simulink model "Model_RL_s"  (R2023a)
settings: Solver=VariableStepAuto  StartTime=0.0  StopTime=20  MaxStep=0.002  RelTol=1e-6
StopFcn:
  | save_run_results('RL', 'manual_run')
values from neighbouring files (symbols this model uses):
  C_r = maskInitContext.MaskWorkspace.get('C_r')    [Mask_bike.m]
  F_zf = m_ * g_ * l_r_ / (l_f_ + l_r_)    [load_derived.m]
  F_zr = m_ * g_ * l_f_ / (l_f_ + l_r_)    [load_derived.m]
  l_f = maskInitContext.MaskWorkspace.get('l_f')    [Mask_Pacejka.m]    (also in Mask_bike.m)
  l_r = maskInitContext.MaskWorkspace.get('l_r')    [Mask_bike.m]
  m = maskInitContext.MaskWorkspace.get('m')    [Mask_bike.m]
  Tdref_ay_bp_ms2 = raw.fine.ay_breakpoints_g(:)' * 9.81    [load_ref.m]
  Tdref_table = raw.fine.table_Nm'    [load_ref.m]
  Tdref_v_bp_ms = raw.fine.v_breakpoints_kmh(:)' / 3.6    [load_ref.m]
undefined symbols (not defined in the file or in its folder): c, C, C_alpha_f, C_col, E, e_c, Iz, J_col, K, n_st, noise_seed_a_y, noise_seed_gamma, noise_seed_T_s, noise_seed_theta1, noise_seed_theta2_dot, noise_seed_v, noise_var_a_y, noise_var_gamma, noise_var_T_s, noise_var_theta1, noise_var_theta2_dot, noise_var_v, rl_done_eT, rl_hist_stride, rl_I_decay, rl_I_gain, rl_I_in, rl_obs_gain, rl_reward_par, rl_Ta_gain, rl_Ts, rl_use_agent, sens_Tupd_a_y, sens_Tupd_gamma, sens_Tupd_T_s, sens_Tupd_theta1, sens_Tupd_theta2_dot, sens_Tupd_v, sensors_on, t_0, T_f, Tamax_table, Tamax_v_bp_ms
libraries: rllib x1
settings Model: Creator=Tan_Tram  LastModifiedBy=Tan_Tram
settings DataIOCC: ReturnWorkspaceOutputs=off

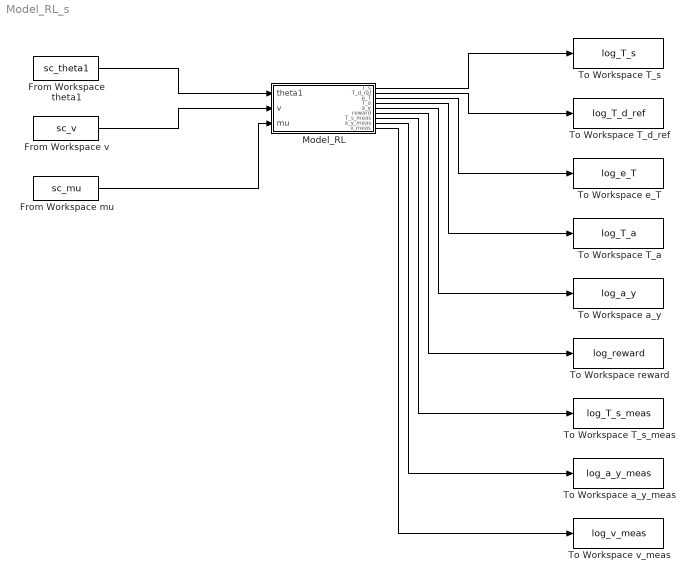
== system Model_RL_s ==
  From Workspace mu : FromWorkspace  VariableName=sc_mu  OutputAfterFinalValue=Holding final value
  From Workspace theta1 : FromWorkspace  VariableName=sc_theta1  OutputAfterFinalValue=Holding final value
  From Workspace v : FromWorkspace  VariableName=sc_v  OutputAfterFinalValue=Holding final value
  Model_RL : Subsystem
  To Workspace T_a : ToWorkspace  VariableName=log_T_a  SaveFormat=Timeseries  SampleTime=-1
  To Workspace T_d_ref : ToWorkspace  VariableName=log_T_d_ref  SaveFormat=Timeseries  SampleTime=-1
  To Workspace T_s : ToWorkspace  VariableName=log_T_s  SaveFormat=Timeseries  SampleTime=-1
  To Workspace T_s_meas : ToWorkspace  VariableName=log_T_s_meas  SaveFormat=Timeseries  SampleTime=-1
  To Workspace a_y : ToWorkspace  VariableName=log_a_y  SaveFormat=Timeseries  SampleTime=-1
  To Workspace a_y_meas : ToWorkspace  VariableName=log_a_y_meas  SaveFormat=Timeseries  SampleTime=-1
  To Workspace e_T : ToWorkspace  VariableName=log_e_T  SaveFormat=Timeseries  SampleTime=-1
  To Workspace reward : ToWorkspace  VariableName=log_reward  SaveFormat=Timeseries  SampleTime=-1
  To Workspace v_meas : ToWorkspace  VariableName=log_v_meas  SaveFormat=Timeseries  SampleTime=-1
  wires:
  From Workspace theta1/1 -> Model_RL/1(theta1)
  From Workspace v/1 -> Model_RL/2(v)
  From Workspace mu/1 -> Model_RL/3(mu)
  Model_RL/1(T_s) -> To Workspace T_s/1
  Model_RL/2(T_d_ref) -> To Workspace T_d_ref/1
  Model_RL/3(e_T) -> To Workspace e_T/1
  Model_RL/4(T_a) -> To Workspace T_a/1
  Model_RL/5(a_y) -> To Workspace a_y/1
  Model_RL/6(reward) -> To Workspace reward/1
  Model_RL/7(T_s_meas) -> To Workspace T_s_meas/1
  Model_RL/8(a_y_meas) -> To Workspace a_y_meas/1
  Model_RL/9(v_meas) -> To Workspace v_meas/1

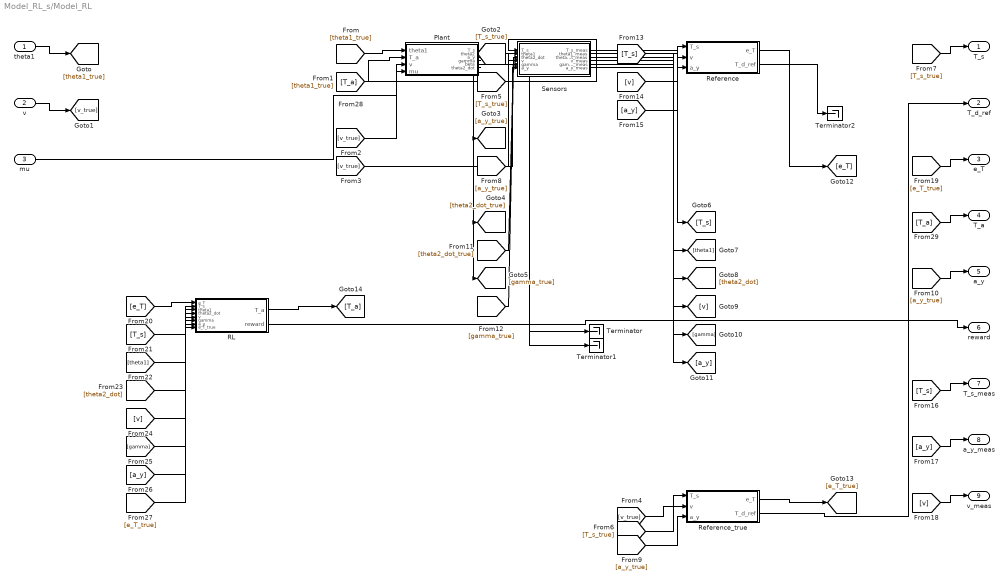
== system Model_RL_s/Model_RL ==
  theta1 : Inport
  v : Inport  Port=2
  mu : Inport  Port=3
  Plant : Subsystem
  RL : Subsystem
  Reference : Subsystem
  Reference_true : Subsystem
  Sensors : Subsystem
  Terminator : Terminator
  Terminator1 : Terminator
  Terminator2 : Terminator
  T_s : Outport
  T_d_ref : Outport  Port=2
  e_T : Outport  Port=3
  T_a : Outport  Port=4
  a_y : Outport  Port=5
  reward : Outport  Port=6
  T_s_meas : Outport  Port=7
  a_y_meas : Outport  Port=8
  v_meas : Outport  Port=9
  wires:
  theta1/1 -> [theta1_true]
  [theta1_true] -> Plant/1(theta1)
  [theta1_true] -> Sensors/2(theta1)
  v/1 -> [v_true]
  [v_true] -> Plant/3(v)
  [v_true] -> Sensors/4(v)
  [v_true] -> Reference_true/2(v)
  mu/1 -> Plant/4(mu)
  Plant/1(T_s) -> [T_s_true]
  [T_s_true] -> Sensors/1(T_s)
  [T_s_true] -> Reference_true/1(T_s)
  [T_s_true] -> T_s/1
  Plant/3(a_y) -> [a_y_true]
  [a_y_true] -> Sensors/6(a_y)
  [a_y_true] -> Reference_true/3(a_y)
  [a_y_true] -> a_y/1
  Plant/6(theta2_dot) -> [theta2_dot_true]
  [theta2_dot_true] -> Sensors/3(theta2_dot)
  Plant/4(gamma) -> [gamma_true]
  [gamma_true] -> Sensors/5(gamma)
  Plant/2(theta2) -> Terminator/1
  Plant/5(beta) -> Terminator1/1
  Sensors/1(T_s_meas) -> [T_s]
  Sensors/2(theta1_meas) -> [theta1]
  Sensors/3(theta2_dot_meas) -> [theta2_dot]
  Sensors/4(v_meas) -> [v]
  Sensors/5(gamma_meas) -> [gamma]
  Sensors/6(a_y_meas) -> [a_y]
  [T_s] -> Reference/1(T_s)
  [v] -> Reference/2(v)
  [a_y] -> Reference/3(a_y)
  [T_s] -> T_s_meas/1
  [a_y] -> a_y_meas/1
  [v] -> v_meas/1
  Reference/1(e_T) -> [e_T]
  Reference/2(T_d_ref) -> Terminator2/1
  Reference_true/1(e_T) -> [e_T_true]
  [e_T_true] -> e_T/1
  Reference_true/2(T_d_ref) -> T_d_ref/1
  [e_T] -> RL/1(e_T)
  [T_s] -> RL/2(T_s)
  [theta1] -> RL/3(theta1)
  [theta2_dot] -> RL/4(theta2_dot)
  [v] -> RL/5(v)
  [gamma] -> RL/6(gamma)
  [a_y] -> RL/7(a_y)
  [e_T_true] -> RL/8(e_T_true)
  RL/1(T_a) -> [T_a]
  [T_a] -> Plant/2(T_a)
  [T_a] -> T_a/1
  RL/2(reward) -> reward/1

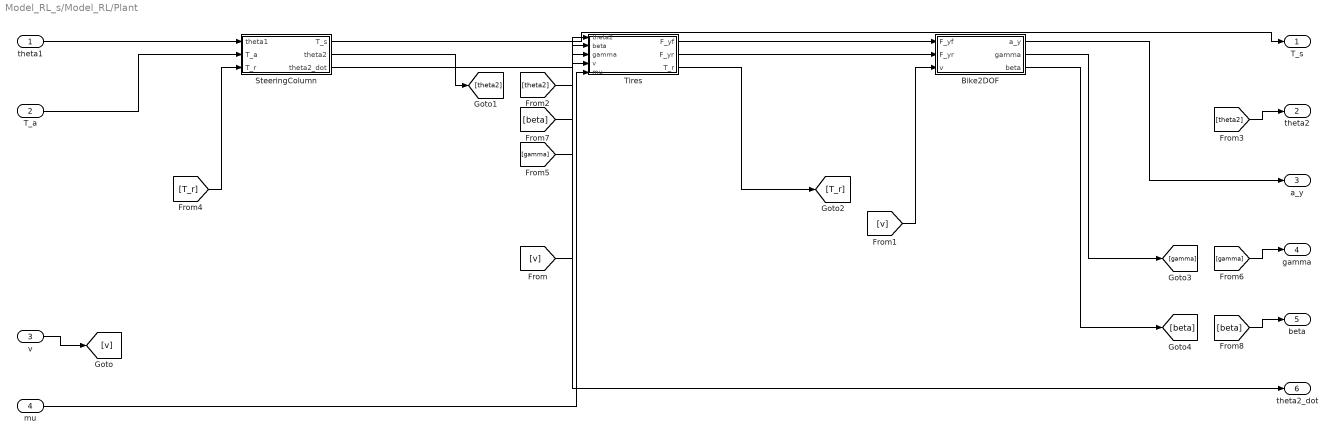
== system Model_RL_s/Model_RL/Plant ==
  theta1 : Inport
  T_a : Inport  Port=2
  v : Inport  Port=3
  mu : Inport  Port=4
  Bike2DOF : Subsystem
  SteeringColumn : Subsystem
  Tires : Subsystem
  T_s : Outport
  theta2 : Outport  Port=2
  a_y : Outport  Port=3
  gamma : Outport  Port=4
  beta : Outport  Port=5
  theta2_dot : Outport  Port=6
  wires:
  [beta] -> beta/1
  [beta] -> Tires/2(beta)
  Bike2DOF/3(beta) -> [beta]
  [gamma] -> gamma/1
  [gamma] -> Tires/3(gamma)
  Bike2DOF/2(gamma) -> [gamma]
  [T_r] -> SteeringColumn/3(T_r)
  Tires/3(T_r) -> [T_r]
  [theta2] -> theta2/1
  [theta2] -> Tires/1(theta2)
  SteeringColumn/2(theta2) -> [theta2]
  [v] -> Bike2DOF/3(v)
  [v] -> Tires/4(v)
  v/1 -> [v]
  SteeringColumn/3(theta2_dot) -> theta2_dot/1
  Bike2DOF/1(a_y) -> a_y/1
  SteeringColumn/1(T_s) -> T_s/1
  Tires/2(F_yr) -> Bike2DOF/2(F_yr)
  Tires/1(F_yf) -> Bike2DOF/1(F_yf)
  mu/1 -> Tires/5(mu)
  T_a/1 -> SteeringColumn/2(T_a)
  theta1/1 -> SteeringColumn/1(theta1)

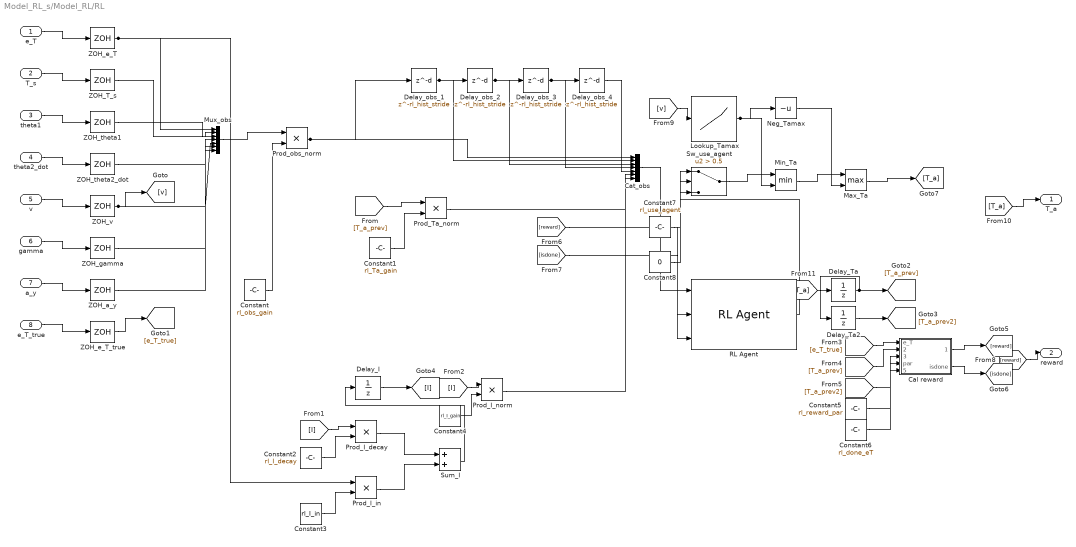
== system Model_RL_s/Model_RL/RL ==
  e_T : Inport
  T_s : Inport  Port=2
  theta1 : Inport  Port=3
  theta2_dot : Inport  Port=4
  v : Inport  Port=5
  gamma : Inport  Port=6
  a_y : Inport  Port=7
  e_T_true : Inport  Port=8
  Cal reward : MATLAB Function  TreatAsAtomicUnit=on
  Cat_obs : Concatenate  NumInputs=7
  Constant : Constant  Value=rl_obs_gain
  Constant1 : Constant  Value=rl_Ta_gain
  Constant2 : Constant  Value=rl_I_decay
  Constant3 : Constant  Value=rl_I_in
  Constant4 : Constant  Value=rl_I_gain
  Constant5 : Constant  Value=rl_reward_par
  Constant6 : Constant  Value=rl_done_eT
  Constant7 : Constant  Value=rl_use_agent
  Constant8 : Constant  Value=0
  Delay_I : UnitDelay  SampleTime=rl_Ts  HasFrameUpgradeWarning=on
  Delay_Ta : UnitDelay  SampleTime=rl_Ts  HasFrameUpgradeWarning=on
  Delay_Ta2 : UnitDelay  SampleTime=rl_Ts  HasFrameUpgradeWarning=on
  Delay_obs_{1..4} (4 alike) : Delay  DelayLength=rl_hist_stride  InitialCondition=0  SampleTime=rl_Ts
  Lookup_Tamax : Lookup_n-D  NumberOfTableDimensions=1  BreakpointsForDimension1=Tamax_v_bp_ms  Table=Tamax_table  ExtrapMethod=Clip  InternalRulePriority=Speed  RndMeth=Simplest
  Max_Ta : MinMax  Function=max  Inputs=2
  Min_Ta : MinMax  Inputs=2
  Mux_obs : Mux  Inputs=7
  Neg_Tamax : UnaryMinus
  Prod_I_decay : Product  Inputs=**
  Prod_I_in : Product  Inputs=**
  Prod_I_norm : Product  Inputs=**
  Prod_Ta_norm : Product  Inputs=**
  Prod_obs_norm : Product  Inputs=**
  RL Agent : rllib/RL Agent  Agent=rl_agent  ExternalActionAsInput=off  ProvideLastAction=off  ProvideCumRwd=off  TreatAsDirectFeedthrough=on  UseStrictObservationDataTypes=off
  Sum_I : Sum
  Sw_use_agent : Switch  Criteria=u2 > Threshold  Threshold=0.5  SaturateOnIntegerOverflow=off  InputSameDT=off
  ZOH_T_s : ZeroOrderHold  SampleTime=rl_Ts
  ZOH_a_y : ZeroOrderHold  SampleTime=rl_Ts
  ZOH_e_T : ZeroOrderHold  SampleTime=rl_Ts
  ZOH_e_T_true : ZeroOrderHold  SampleTime=rl_Ts
  ZOH_gamma : ZeroOrderHold  SampleTime=rl_Ts
  ZOH_theta1 : ZeroOrderHold  SampleTime=rl_Ts
  ZOH_theta2_dot : ZeroOrderHold  SampleTime=rl_Ts
  ZOH_v : ZeroOrderHold  SampleTime=rl_Ts
  T_a : Outport
  reward : Outport  Port=2
  wires:
  e_T/1 -> ZOH_e_T/1
  T_s/1 -> ZOH_T_s/1
  theta1/1 -> ZOH_theta1/1
  theta2_dot/1 -> ZOH_theta2_dot/1
  v/1 -> ZOH_v/1
  ZOH_v/1 -> [v], Mux_obs/5
  gamma/1 -> ZOH_gamma/1
  a_y/1 -> ZOH_a_y/1
  e_T_true/1 -> ZOH_e_T_true/1
  ZOH_e_T_true/1 -> [e_T_true]
  ZOH_e_T/1 -> Mux_obs/1, Prod_I_in/1
  ZOH_T_s/1 -> Mux_obs/2
  ZOH_theta1/1 -> Mux_obs/3
  ZOH_theta2_dot/1 -> Mux_obs/4
  ZOH_gamma/1 -> Mux_obs/6
  ZOH_a_y/1 -> Mux_obs/7
  Mux_obs/1 -> Prod_obs_norm/1
  Constant/1 -> Prod_obs_norm/2
  Prod_obs_norm/1 -> Delay_obs_1/1, Cat_obs/1
  Delay_obs_1/1 -> Delay_obs_2/1, Cat_obs/2
  Delay_obs_2/1 -> Delay_obs_3/1, Cat_obs/3
  Delay_obs_3/1 -> Delay_obs_4/1, Cat_obs/4
  Delay_Ta/1 -> [T_a_prev], Delay_Ta2/1
  Delay_Ta2/1 -> [T_a_prev2]
  [T_a_prev] -> Prod_Ta_norm/1
  Constant1/1 -> Prod_Ta_norm/2
  Delay_I/1 -> [I]
  [I] -> Prod_I_decay/1
  Constant2/1 -> Prod_I_decay/2
  Constant3/1 -> Prod_I_in/2
  Prod_I_decay/1 -> Sum_I/1
  Prod_I_in/1 -> Sum_I/2
  Sum_I/1 -> Delay_I/1
  [I] -> Prod_I_norm/1
  Constant4/1 -> Prod_I_norm/2
  Delay_obs_4/1 -> Cat_obs/5
  Prod_Ta_norm/1 -> Cat_obs/6
  Prod_I_norm/1 -> Cat_obs/7
  Cat_obs/1 -> RL Agent/1
  [e_T_true] -> Cal reward/1(e_T)
  [T_a_prev] -> Cal reward/2(T_a_prev)
  [T_a_prev2] -> Cal reward/3(T_a_prev2)
  Constant5/1 -> Cal reward/4(par)
  Constant6/1 -> Cal reward/5(done_eT)
  Cal reward/1(reward) -> [reward]
  Cal reward/2(isdone) -> [isdone]
  [reward] -> RL Agent/2
  [isdone] -> RL Agent/3
  [reward] -> reward/1
  RL Agent/1 -> Sw_use_agent/1
  Constant7/1 -> Sw_use_agent/2
  Constant8/1 -> Sw_use_agent/3
  [v] -> Lookup_Tamax/1
  Sw_use_agent/1 -> Min_Ta/1
  Lookup_Tamax/1 -> Min_Ta/2, Neg_Tamax/1
  Min_Ta/1 -> Max_Ta/1
  Neg_Tamax/1 -> Max_Ta/2
  Max_Ta/1 -> [T_a]
  [T_a] -> T_a/1
  [T_a] -> Delay_Ta/1

== system Model_RL_s/Model_RL/Reference ==
  T_s : Inport
  v : Inport  Port=2
  a_y : Inport  Port=3
  Cal T_d_ref : Subsystem
  Sum_eT : Sum  Inputs=+-
  e_T : Outport
  T_d_ref : Outport  Port=2
  wires:
  Sum_eT/1 -> e_T/1
  T_s/1 -> Sum_eT/1
  [T_d_ref] -> T_d_ref/1
  [T_d_ref] -> Sum_eT/2
  Cal T_d_ref/1(T_d_ref) -> [T_d_ref]
  a_y/1 -> Cal T_d_ref/2(a_y)
  v/1 -> Cal T_d_ref/1(v)

== system Model_RL_s/Model_RL/Reference_true ==
  T_s : Inport
  v : Inport  Port=2
  a_y : Inport  Port=3
  Cal T_d_ref : Subsystem
  Sum_eT : Sum  Inputs=+-
  e_T : Outport
  T_d_ref : Outport  Port=2
  wires:
  Sum_eT/1 -> e_T/1
  T_s/1 -> Sum_eT/1
  [T_d_ref] -> T_d_ref/1
  [T_d_ref] -> Sum_eT/2
  Cal T_d_ref/1(T_d_ref) -> [T_d_ref]
  a_y/1 -> Cal T_d_ref/2(a_y)
  v/1 -> Cal T_d_ref/1(v)

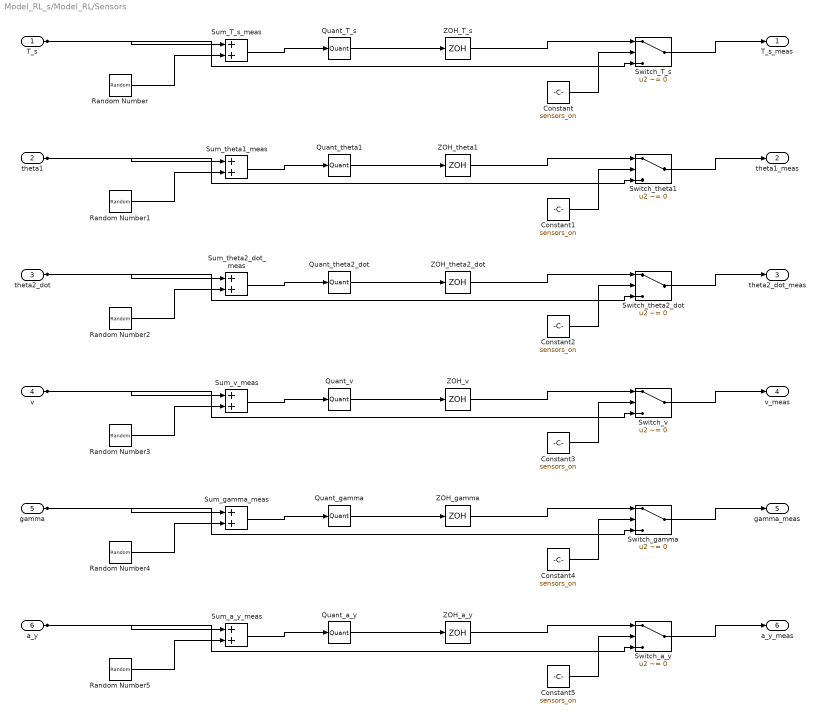
== system Model_RL_s/Model_RL/Sensors ==
  T_s : Inport
  theta1 : Inport  Port=2
  theta2_dot : Inport  Port=3
  v : Inport  Port=4
  gamma : Inport  Port=5
  a_y : Inport  Port=6
  Constant{,1..5} (6 alike) : Constant  Value=sensors_on
  Quant_T_s : Quantizer  QuantizationInterval=sens_delta_T_s
  Quant_a_y : Quantizer  QuantizationInterval=sens_delta_a_y
  Quant_gamma : Quantizer  QuantizationInterval=sens_delta_gamma
  Quant_theta1 : Quantizer  QuantizationInterval=sens_delta_theta1
  Quant_theta2_dot : Quantizer  QuantizationInterval=sens_delta_theta2_dot
  Quant_v : Quantizer  QuantizationInterval=sens_delta_v
  Random Number : RandomNumber  Variance=noise_var_T_s  Seed=noise_seed_T_s  SampleTime=sens_Tupd_T_s
  Random Number1 : RandomNumber  Variance=noise_var_theta1  Seed=noise_seed_theta1  SampleTime=sens_Tupd_theta1
  Random Number2 : RandomNumber  Variance=noise_var_theta2_dot  Seed=noise_seed_theta2_dot  SampleTime=sens_Tupd_theta2_dot
  Random Number3 : RandomNumber  Variance=noise_var_v  Seed=noise_seed_v  SampleTime=sens_Tupd_v
  Random Number4 : RandomNumber  Variance=noise_var_gamma  Seed=noise_seed_gamma  SampleTime=sens_Tupd_gamma
  Random Number5 : RandomNumber  Variance=noise_var_a_y  Seed=noise_seed_a_y  SampleTime=sens_Tupd_a_y
  Sum_T_s_meas : Sum
  Sum_a_y_meas : Sum
  Sum_gamma_meas : Sum
  Sum_theta1_meas : Sum
  Sum_theta2_dot_meas : Sum
  Sum_v_meas : Sum
  Switch_T_s : Switch  Criteria=u2 ~= 0  SaturateOnIntegerOverflow=off  InputSameDT=off
  Switch_a_y : Switch  Criteria=u2 ~= 0  SaturateOnIntegerOverflow=off  InputSameDT=off
  Switch_gamma : Switch  Criteria=u2 ~= 0  SaturateOnIntegerOverflow=off  InputSameDT=off
  Switch_theta1 : Switch  Criteria=u2 ~= 0  SaturateOnIntegerOverflow=off  InputSameDT=off
  Switch_theta2_dot : Switch  Criteria=u2 ~= 0  SaturateOnIntegerOverflow=off  InputSameDT=off
  Switch_v : Switch  Criteria=u2 ~= 0  SaturateOnIntegerOverflow=off  InputSameDT=off
  ZOH_T_s : ZeroOrderHold  SampleTime=sens_Tupd_T_s
  ZOH_a_y : ZeroOrderHold  SampleTime=sens_Tupd_a_y
  ZOH_gamma : ZeroOrderHold  SampleTime=sens_Tupd_gamma
  ZOH_theta1 : ZeroOrderHold  SampleTime=sens_Tupd_theta1
  ZOH_theta2_dot : ZeroOrderHold  SampleTime=sens_Tupd_theta2_dot
  ZOH_v : ZeroOrderHold  SampleTime=sens_Tupd_v
  T_s_meas : Outport
  theta1_meas : Outport  Port=2
  theta2_dot_meas : Outport  Port=3
  v_meas : Outport  Port=4
  gamma_meas : Outport  Port=5
  a_y_meas : Outport  Port=6
  wires:
  T_s/1 -> Sum_T_s_meas/1, Switch_T_s/3
  Random Number/1 -> Sum_T_s_meas/2
  Sum_T_s_meas/1 -> Quant_T_s/1
  Quant_T_s/1 -> ZOH_T_s/1
  ZOH_T_s/1 -> Switch_T_s/1
  Constant/1 -> Switch_T_s/2
  Switch_T_s/1 -> T_s_meas/1
  theta1/1 -> Sum_theta1_meas/1, Switch_theta1/3
  Random Number1/1 -> Sum_theta1_meas/2
  Sum_theta1_meas/1 -> Quant_theta1/1
  Quant_theta1/1 -> ZOH_theta1/1
  ZOH_theta1/1 -> Switch_theta1/1
  Constant1/1 -> Switch_theta1/2
  Switch_theta1/1 -> theta1_meas/1
  theta2_dot/1 -> Sum_theta2_dot_meas/1, Switch_theta2_dot/3
  Random Number2/1 -> Sum_theta2_dot_meas/2
  Sum_theta2_dot_meas/1 -> Quant_theta2_dot/1
  Quant_theta2_dot/1 -> ZOH_theta2_dot/1
  ZOH_theta2_dot/1 -> Switch_theta2_dot/1
  Constant2/1 -> Switch_theta2_dot/2
  Switch_theta2_dot/1 -> theta2_dot_meas/1
  v/1 -> Sum_v_meas/1, Switch_v/3
  Random Number3/1 -> Sum_v_meas/2
  Sum_v_meas/1 -> Quant_v/1
  Quant_v/1 -> ZOH_v/1
  ZOH_v/1 -> Switch_v/1
  Constant3/1 -> Switch_v/2
  Switch_v/1 -> v_meas/1
  gamma/1 -> Sum_gamma_meas/1, Switch_gamma/3
  Random Number4/1 -> Sum_gamma_meas/2
  Sum_gamma_meas/1 -> Quant_gamma/1
  Quant_gamma/1 -> ZOH_gamma/1
  ZOH_gamma/1 -> Switch_gamma/1
  Constant4/1 -> Switch_gamma/2
  Switch_gamma/1 -> gamma_meas/1
  a_y/1 -> Sum_a_y_meas/1, Switch_a_y/3
  Random Number5/1 -> Sum_a_y_meas/2
  Sum_a_y_meas/1 -> Quant_a_y/1
  Quant_a_y/1 -> ZOH_a_y/1
  ZOH_a_y/1 -> Switch_a_y/1
  Constant5/1 -> Switch_a_y/2
  Switch_a_y/1 -> a_y_meas/1

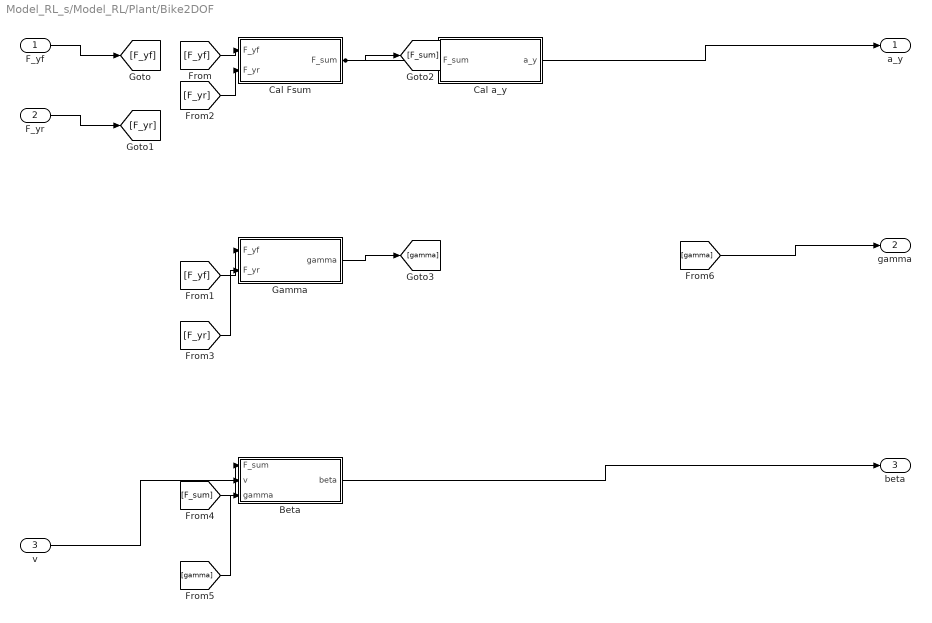
== system Model_RL_s/Model_RL/Plant/Bike2DOF ==
  F_yf : Inport
  F_yr : Inport  Port=2
  v : Inport  Port=3
  Beta : Subsystem
  Cal Fsum : Subsystem
  Cal a_y : Subsystem
  Gamma : Subsystem
  a_y : Outport
  gamma : Outport  Port=2
  beta : Outport  Port=3
  wires:
  F_yf/1 -> [F_yf]
  [F_yf] -> Cal Fsum/1(F_yf)
  [F_yf] -> Gamma/1(F_yf)
  F_yr/1 -> [F_yr]
  [F_yr] -> Cal Fsum/2(F_yr)
  [F_yr] -> Gamma/2(F_yr)
  Cal Fsum/1(F_sum) -> Cal a_y/1(F_sum), [F_sum]
  [F_sum] -> Beta/1(F_sum)
  Cal a_y/1(a_y) -> a_y/1
  Gamma/1(gamma) -> [gamma]
  [gamma] -> Beta/3(gamma)
  [gamma] -> gamma/1
  v/1 -> Beta/2(v)
  Beta/1(beta) -> beta/1

== system Model_RL_s/Model_RL/Plant/SteeringColumn ==
  theta1 : Inport
  T_a : Inport  Port=2
  T_r : Inport  Port=3
  Cal T_s : Subsystem
  Lower : Subsystem
  T_s : Outport
  theta2 : Outport  Port=2
  theta2_dot : Outport  Port=3
  wires:
  theta1/1 -> Cal T_s/1(theta1)
  T_a/1 -> Lower/1(T_a)
  T_r/1 -> Lower/2(T_r)
  Lower/2(theta2_dot) -> theta2_dot/1
  Lower/1(theta2) -> [theta2]
  [theta2] -> Cal T_s/2(theta2)
  [theta2] -> theta2/1
  Cal T_s/1(T_s) -> [T_s]
  [T_s] -> Lower/3(T_s)
  [T_s] -> T_s/1

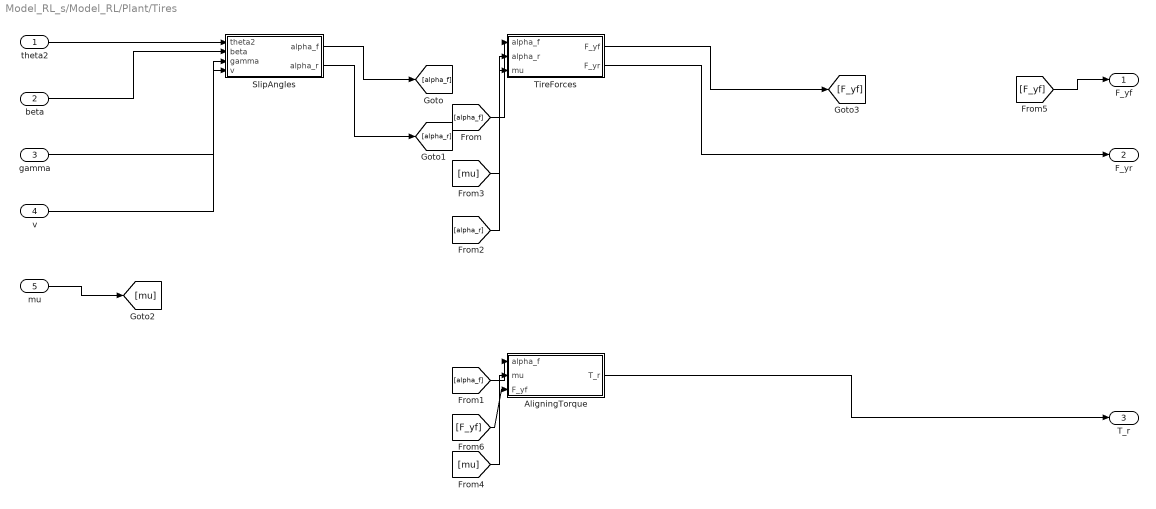
== system Model_RL_s/Model_RL/Plant/Tires ==
  theta2 : Inport
  beta : Inport  Port=2
  gamma : Inport  Port=3
  v : Inport  Port=4
  mu : Inport  Port=5
  AligningTorque : Subsystem
  SlipAngles : Subsystem
  TireForces : Subsystem
  F_yf : Outport
  F_yr : Outport  Port=2
  T_r : Outport  Port=3
  wires:
  theta2/1 -> SlipAngles/1(theta2)
  beta/1 -> SlipAngles/2(beta)
  gamma/1 -> SlipAngles/3(gamma)
  v/1 -> SlipAngles/4(v)
  SlipAngles/1(alpha_f) -> [alpha_f]
  [alpha_f] -> TireForces/1(alpha_f)
  [alpha_f] -> AligningTorque/1(alpha_f)
  SlipAngles/2(alpha_r) -> [alpha_r]
  [alpha_r] -> TireForces/2(alpha_r)
  mu/1 -> [mu]
  [mu] -> TireForces/3(mu)
  [mu] -> AligningTorque/2(mu)
  TireForces/1(F_yf) -> [F_yf]
  [F_yf] -> F_yf/1
  [F_yf] -> AligningTorque/3(F_yf)
  TireForces/2(F_yr) -> F_yr/1
  AligningTorque/1(T_r) -> T_r/1

== system Model_RL_s/Model_RL/Reference/Cal T_d_ref ==
  v : Inport
  a_y : Inport  Port=2
  Abs_ay : Abs  SaturateOnIntegerOverflow=off
  LUT_Tdref : Lookup_n-D  BreakpointsForDimension1=Tdref_v_bp_ms  BreakpointsForDimension2=Tdref_ay_bp_ms2  Table=Tdref_table  ExtrapMethod=Clip  InternalRulePriority=Speed  RndMeth=Simplest
      settings: InputPortMap=u0,u1
  Prod_Tdref : Product  Inputs=**
  Sign_ay : Signum
  T_d_ref : Outport
  wires:
  Prod_Tdref/1 -> T_d_ref/1
  Sign_ay/1 -> Prod_Tdref/2
  LUT_Tdref/1 -> Prod_Tdref/1
  [a_y] -> Sign_ay/1
  Abs_ay/1 -> LUT_Tdref/2
  [a_y] -> Abs_ay/1
  v/1 -> LUT_Tdref/1
  a_y/1 -> [a_y]

== system Model_RL_s/Model_RL/Reference_true/Cal T_d_ref ==
  v : Inport
  a_y : Inport  Port=2
  Abs_ay : Abs  SaturateOnIntegerOverflow=off
  LUT_Tdref : Lookup_n-D  BreakpointsForDimension1=Tdref_v_bp_ms  BreakpointsForDimension2=Tdref_ay_bp_ms2  Table=Tdref_table  ExtrapMethod=Clip  InternalRulePriority=Speed  RndMeth=Simplest
      settings: InputPortMap=u0,u1
  Prod_Tdref : Product  Inputs=**
  Sign_ay : Signum
  T_d_ref : Outport
  wires:
  Prod_Tdref/1 -> T_d_ref/1
  Sign_ay/1 -> Prod_Tdref/2
  LUT_Tdref/1 -> Prod_Tdref/1
  [a_y] -> Sign_ay/1
  Abs_ay/1 -> LUT_Tdref/2
  [a_y] -> Abs_ay/1
  v/1 -> LUT_Tdref/1
  a_y/1 -> [a_y]

== system Model_RL_s/Model_RL/Plant/Bike2DOF/Beta ==
  F_sum : Inport
  v : Inport  Port=2
  gamma : Inport  Port=3
  Constant : Constant  Value=m
  Div_Fsum_mv : Product  Inputs=*/
  Int_beta : Integrator
  Prod_mv : Product  Inputs=**
  Sum_betadot : Sum  Inputs=+-
  beta : Outport
  wires:
  Constant/1 -> Prod_mv/1
  v/1 -> Prod_mv/2
  F_sum/1 -> Div_Fsum_mv/1
  Prod_mv/1 -> Div_Fsum_mv/2
  Div_Fsum_mv/1 -> Sum_betadot/1
  gamma/1 -> Sum_betadot/2
  Sum_betadot/1 -> Int_beta/1
  Int_beta/1 -> beta/1

== system Model_RL_s/Model_RL/Plant/Bike2DOF/Cal Fsum ==
  F_yf : Inport
  F_yr : Inport  Port=2
  Sum_Fsum : Sum
  F_sum : Outport
  wires:
  F_yf/1 -> Sum_Fsum/1
  F_yr/1 -> Sum_Fsum/2
  Sum_Fsum/1 -> F_sum/1

== system Model_RL_s/Model_RL/Plant/Bike2DOF/Cal a_y ==
  F_sum : Inport
  Constant : Constant  Value=m
  Div_ay : Product  Inputs=*/
  a_y : Outport
  wires:
  F_sum/1 -> Div_ay/1
  Constant/1 -> Div_ay/2
  Div_ay/1 -> a_y/1

== system Model_RL_s/Model_RL/Plant/Bike2DOF/Gamma ==
  F_yf : Inport
  F_yr : Inport  Port=2
  Constant : Constant  Value=l_f
  Constant1 : Constant  Value=l_r
  Constant2 : Constant  Value=Iz
  Div_gammadot : Product  Inputs=*/
  Int_gamma : Integrator
  Prod_lfFyf : Product  Inputs=**
  Prod_lrFyr : Product  Inputs=**
  Sum_moment : Sum  Inputs=+-
  gamma : Outport
  wires:
  Constant/1 -> Prod_lfFyf/1
  F_yf/1 -> Prod_lfFyf/2
  Constant1/1 -> Prod_lrFyr/1
  F_yr/1 -> Prod_lrFyr/2
  Prod_lfFyf/1 -> Sum_moment/1
  Prod_lrFyr/1 -> Sum_moment/2
  Sum_moment/1 -> Div_gammadot/1
  Constant2/1 -> Div_gammadot/2
  Div_gammadot/1 -> Int_gamma/1
  Int_gamma/1 -> gamma/1

== system Model_RL_s/Model_RL/Plant/SteeringColumn/Cal T_s ==
  theta1 : Inport
  theta2 : Inport  Port=2
  Constant : Constant  Value=K
  Prod_Ts : Product  Inputs=**
  Sum_dTheta : Sum  Inputs=+-
  T_s : Outport
  wires:
  theta1/1 -> Sum_dTheta/1
  theta2/1 -> Sum_dTheta/2
  Sum_dTheta/1 -> Prod_Ts/1
  Constant/1 -> Prod_Ts/2
  Prod_Ts/1 -> T_s/1

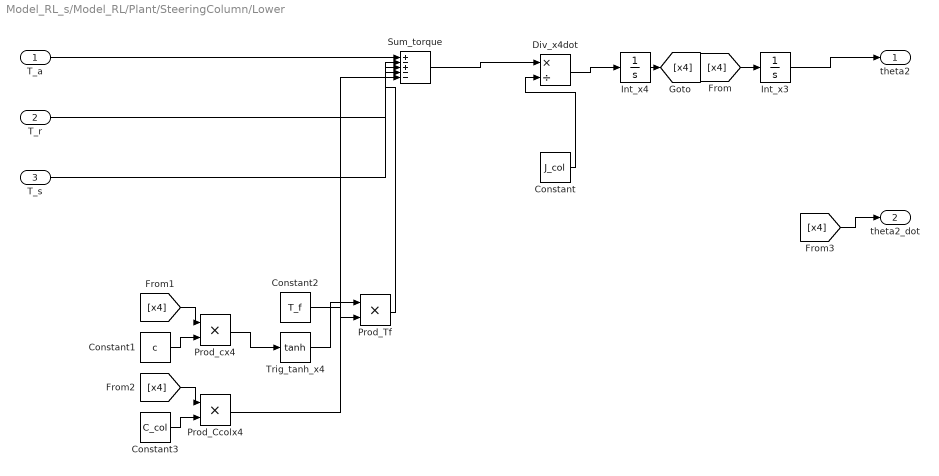
== system Model_RL_s/Model_RL/Plant/SteeringColumn/Lower ==
  T_a : Inport
  T_r : Inport  Port=2
  T_s : Inport  Port=3
  Constant : Constant  Value=J_col
  Constant1 : Constant  Value=c
  Constant2 : Constant  Value=T_f
  Constant3 : Constant  Value=C_col
  Div_x4dot : Product  Inputs=*/
  Int_x3 : Integrator
  Int_x4 : Integrator
  Prod_Ccolx4 : Product  Inputs=**
  Prod_Tf : Product  Inputs=**
  Prod_cx4 : Product  Inputs=**
  Sum_torque : Sum  Inputs=+-+--
  Trig_tanh_x4 : Trigonometry  Operator=tanh
  theta2 : Outport
  theta2_dot : Outport  Port=2
  wires:
  Int_x4/1 -> [x4]
  [x4] -> Prod_cx4/1
  Constant1/1 -> Prod_cx4/2
  Prod_cx4/1 -> Trig_tanh_x4/1
  Trig_tanh_x4/1 -> Prod_Tf/1
  Constant2/1 -> Prod_Tf/2
  [x4] -> Prod_Ccolx4/1
  Constant3/1 -> Prod_Ccolx4/2
  T_a/1 -> Sum_torque/1
  T_r/1 -> Sum_torque/2
  T_s/1 -> Sum_torque/3
  Prod_Tf/1 -> Sum_torque/4
  Prod_Ccolx4/1 -> Sum_torque/5
  Sum_torque/1 -> Div_x4dot/1
  Constant/1 -> Div_x4dot/2
  Div_x4dot/1 -> Int_x4/1
  [x4] -> Int_x3/1
  Int_x3/1 -> theta2/1
  [x4] -> theta2_dot/1

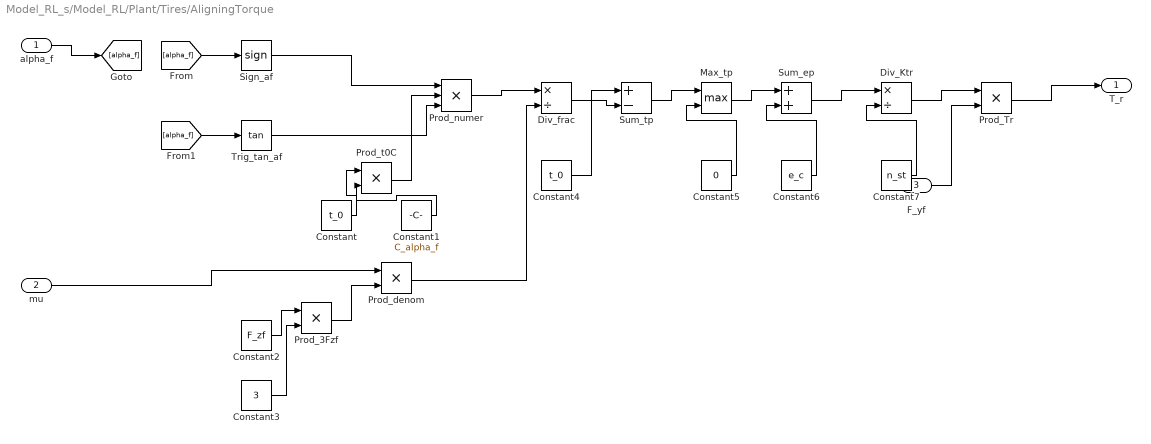
== system Model_RL_s/Model_RL/Plant/Tires/AligningTorque ==
  alpha_f : Inport
  mu : Inport  Port=2
  F_yf : Inport  Port=3
  Constant : Constant  Value=t_0
  Constant1 : Constant  Value=C_alpha_f
  Constant2 : Constant  Value=F_zf
  Constant3 : Constant  Value=3
  Constant4 : Constant  Value=t_0
  Constant5 : Constant  Value=0
  Constant6 : Constant  Value=e_c
  Constant7 : Constant  Value=n_st
  Div_Ktr : Product  Inputs=*/
  Div_frac : Product  Inputs=*/
  Max_tp : MinMax  Function=max  Inputs=2
  Prod_3Fzf : Product  Inputs=**
  Prod_Tr : Product  Inputs=**
  Prod_denom : Product  Inputs=**
  Prod_numer : Product  Inputs=***
  Prod_t0C : Product  Inputs=**
  Sign_af : Signum
  Sum_ep : Sum
  Sum_tp : Sum  Inputs=+-
  Trig_tan_af : Trigonometry  Operator=tan
  T_r : Outport
  wires:
  alpha_f/1 -> [alpha_f]
  [alpha_f] -> Sign_af/1
  [alpha_f] -> Trig_tan_af/1
  Constant/1 -> Prod_t0C/1
  Constant1/1 -> Prod_t0C/2
  Sign_af/1 -> Prod_numer/1
  Prod_t0C/1 -> Prod_numer/2
  Trig_tan_af/1 -> Prod_numer/3
  Constant2/1 -> Prod_3Fzf/1
  Constant3/1 -> Prod_3Fzf/2
  mu/1 -> Prod_denom/1
  Prod_3Fzf/1 -> Prod_denom/2
  Prod_numer/1 -> Div_frac/1
  Prod_denom/1 -> Div_frac/2
  Constant4/1 -> Sum_tp/1
  Div_frac/1 -> Sum_tp/2
  Sum_tp/1 -> Max_tp/1
  Constant5/1 -> Max_tp/2
  Max_tp/1 -> Sum_ep/1
  Constant6/1 -> Sum_ep/2
  Sum_ep/1 -> Div_Ktr/1
  Constant7/1 -> Div_Ktr/2
  Div_Ktr/1 -> Prod_Tr/1
  F_yf/1 -> Prod_Tr/2
  Prod_Tr/1 -> T_r/1

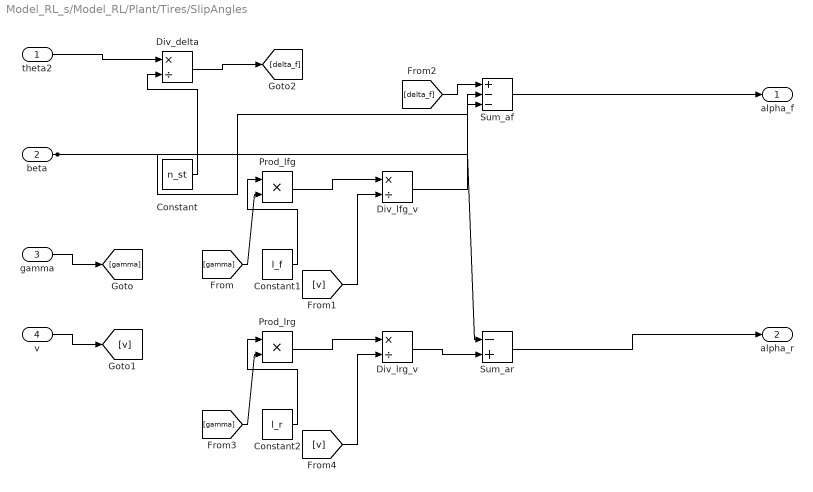
== system Model_RL_s/Model_RL/Plant/Tires/SlipAngles ==
  theta2 : Inport
  beta : Inport  Port=2
  gamma : Inport  Port=3
  v : Inport  Port=4
  Constant : Constant  Value=n_st
  Constant1 : Constant  Value=l_f
  Constant2 : Constant  Value=l_r
  Div_delta : Product  Inputs=*/
  Div_lfg_v : Product  Inputs=*/
  Div_lrg_v : Product  Inputs=*/
  Prod_lfg : Product  Inputs=**
  Prod_lrg : Product  Inputs=**
  Sum_af : Sum  Inputs=+--
  Sum_ar : Sum  Inputs=-+
  alpha_f : Outport
  alpha_r : Outport  Port=2
  wires:
  gamma/1 -> [gamma]
  v/1 -> [v]
  theta2/1 -> Div_delta/1
  Constant/1 -> Div_delta/2
  Constant1/1 -> Prod_lfg/1
  [gamma] -> Prod_lfg/2
  Prod_lfg/1 -> Div_lfg_v/1
  [v] -> Div_lfg_v/2
  Div_delta/1 -> [delta_f]
  [delta_f] -> Sum_af/1
  beta/1 -> Sum_af/2, Sum_ar/1
  Div_lfg_v/1 -> Sum_af/3
  Sum_af/1 -> alpha_f/1
  Constant2/1 -> Prod_lrg/1
  [gamma] -> Prod_lrg/2
  Prod_lrg/1 -> Div_lrg_v/1
  [v] -> Div_lrg_v/2
  Div_lrg_v/1 -> Sum_ar/2
  Sum_ar/1 -> alpha_r/1

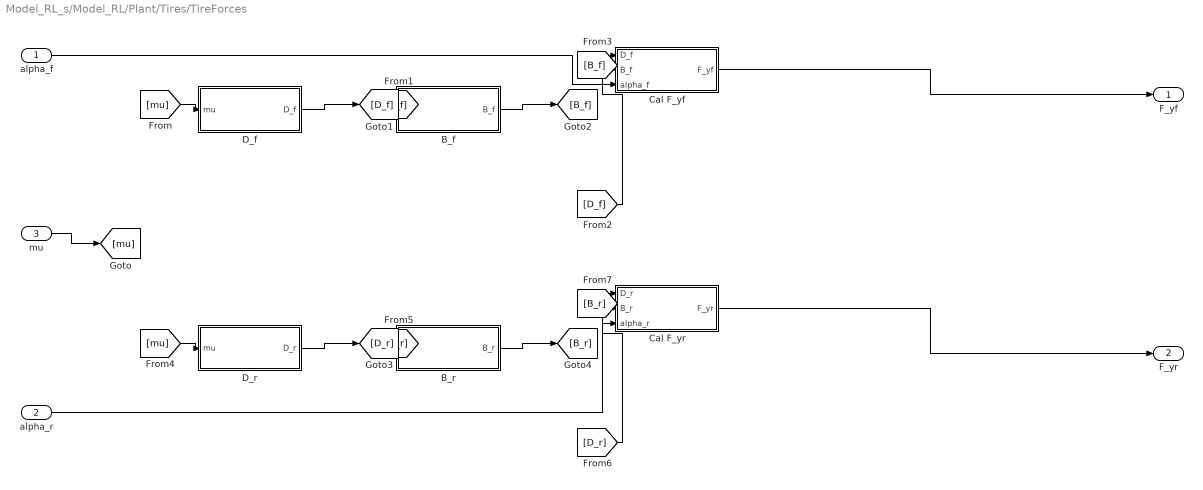
== system Model_RL_s/Model_RL/Plant/Tires/TireForces ==
  alpha_f : Inport
  alpha_r : Inport  Port=2
  mu : Inport  Port=3
  B_f : Subsystem
  B_r : Subsystem
  Cal F_yf : Subsystem
  Cal F_yr : Subsystem
  D_f : Subsystem
  D_r : Subsystem
  F_yf : Outport
  F_yr : Outport  Port=2
  wires:
  mu/1 -> [mu]
  [mu] -> D_f/1(mu)
  D_f/1(D_f) -> [D_f]
  [D_f] -> B_f/1(D_f)
  [D_f] -> Cal F_yf/1(D_f)
  B_f/1(B_f) -> [B_f]
  [B_f] -> Cal F_yf/2(B_f)
  alpha_f/1 -> Cal F_yf/3(alpha_f)
  Cal F_yf/1(F_yf) -> F_yf/1
  [mu] -> D_r/1(mu)
  D_r/1(D_r) -> [D_r]
  [D_r] -> B_r/1(D_r)
  [D_r] -> Cal F_yr/1(D_r)
  B_r/1(B_r) -> [B_r]
  [B_r] -> Cal F_yr/2(B_r)
  alpha_r/1 -> Cal F_yr/3(alpha_r)
  Cal F_yr/1(F_yr) -> F_yr/1

== system Model_RL_s/Model_RL/Plant/Tires/TireForces/B_f ==
  D_f : Inport
  Constant : Constant  Value=C
  Constant1 : Constant  Value=C_alpha_f
  Div_B : Product  Inputs=*/
  Prod_CD : Product  Inputs=**
  B_f : Outport
  wires:
  D_f/1 -> Prod_CD/1
  Constant/1 -> Prod_CD/2
  Constant1/1 -> Div_B/1
  Prod_CD/1 -> Div_B/2
  Div_B/1 -> B_f/1

== system Model_RL_s/Model_RL/Plant/Tires/TireForces/B_r ==
  D_r : Inport
  Constant : Constant  Value=C
  Constant1 : Constant  Value=C_r
  Div_B : Product  Inputs=*/
  Prod_CD : Product  Inputs=**
  B_r : Outport
  wires:
  D_r/1 -> Prod_CD/1
  Constant/1 -> Prod_CD/2
  Constant1/1 -> Div_B/1
  Prod_CD/1 -> Div_B/2
  Div_B/1 -> B_r/1

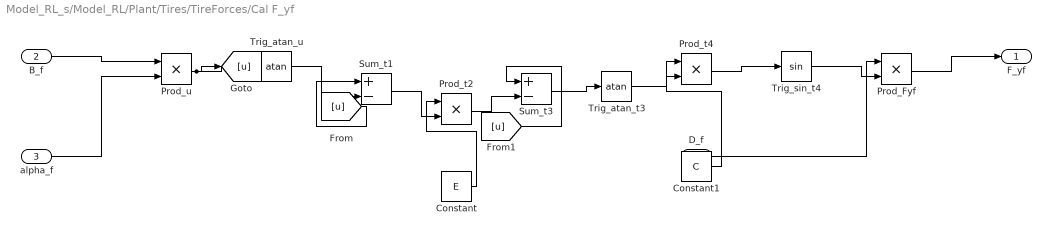
== system Model_RL_s/Model_RL/Plant/Tires/TireForces/Cal F_yf ==
  D_f : Inport
  B_f : Inport  Port=2
  alpha_f : Inport  Port=3
  Constant : Constant  Value=E
  Constant1 : Constant  Value=C
  Prod_Fyf : Product  Inputs=**
  Prod_t2 : Product  Inputs=**
  Prod_t4 : Product  Inputs=**
  Prod_u : Product  Inputs=**
  Sum_t1 : Sum  Inputs=+-
  Sum_t3 : Sum  Inputs=+-
  Trig_atan_t3 : Trigonometry  Operator=atan
  Trig_atan_u : Trigonometry  Operator=atan
  Trig_sin_t4 : Trigonometry
  F_yf : Outport
  wires:
  B_f/1 -> Prod_u/1
  alpha_f/1 -> Prod_u/2
  Prod_u/1 -> Trig_atan_u/1, [u]
  [u] -> Sum_t1/1
  Trig_atan_u/1 -> Sum_t1/2
  Constant/1 -> Prod_t2/1
  Sum_t1/1 -> Prod_t2/2
  [u] -> Sum_t3/1
  Prod_t2/1 -> Sum_t3/2
  Sum_t3/1 -> Trig_atan_t3/1
  Constant1/1 -> Prod_t4/1
  Trig_atan_t3/1 -> Prod_t4/2
  Prod_t4/1 -> Trig_sin_t4/1
  D_f/1 -> Prod_Fyf/1
  Trig_sin_t4/1 -> Prod_Fyf/2
  Prod_Fyf/1 -> F_yf/1

== system Model_RL_s/Model_RL/Plant/Tires/TireForces/Cal F_yr ==
  D_r : Inport
  B_r : Inport  Port=2
  alpha_r : Inport  Port=3
  Constant : Constant  Value=E
  Constant1 : Constant  Value=C
  Prod_Fyr : Product  Inputs=**
  Prod_t2 : Product  Inputs=**
  Prod_t4 : Product  Inputs=**
  Prod_u : Product  Inputs=**
  Sum_t1 : Sum  Inputs=+-
  Sum_t3 : Sum  Inputs=+-
  Trig_atan_t3 : Trigonometry  Operator=atan
  Trig_atan_u : Trigonometry  Operator=atan
  Trig_sin_t4 : Trigonometry
  F_yr : Outport
  wires:
  B_r/1 -> Prod_u/1
  alpha_r/1 -> Prod_u/2
  Prod_u/1 -> Trig_atan_u/1, [u]
  [u] -> Sum_t1/1
  Trig_atan_u/1 -> Sum_t1/2
  Constant/1 -> Prod_t2/1
  Sum_t1/1 -> Prod_t2/2
  [u] -> Sum_t3/1
  Prod_t2/1 -> Sum_t3/2
  Sum_t3/1 -> Trig_atan_t3/1
  Constant1/1 -> Prod_t4/1
  Trig_atan_t3/1 -> Prod_t4/2
  Prod_t4/1 -> Trig_sin_t4/1
  D_r/1 -> Prod_Fyr/1
  Trig_sin_t4/1 -> Prod_Fyr/2
  Prod_Fyr/1 -> F_yr/1

== system Model_RL_s/Model_RL/Plant/Tires/TireForces/D_f ==
  mu : Inport
  Constant : Constant  Value=F_zf
  Prod_D : Product  Inputs=**
  D_f : Outport
  wires:
  mu/1 -> Prod_D/1
  Constant/1 -> Prod_D/2
  Prod_D/1 -> D_f/1

== system Model_RL_s/Model_RL/Plant/Tires/TireForces/D_r ==
  mu : Inport
  Constant : Constant  Value=F_zr
  Prod_D : Product  Inputs=**
  D_r : Outport
  wires:
  mu/1 -> Prod_D/1
  Constant/1 -> Prod_D/2
  Prod_D/1 -> D_r/1

== matlab function Model_RL_s/Model_RL/RL/Cal reward ==
  data: e_T input; reward output; T_a_prev input; T_a_prev2 input; par input; done_eT input; isdone output
function [reward, isdone] = cal_reward(e_T, T_a_prev, T_a_prev2, par, done_eT)
% Step reward of Documents/RL/DieuKhien_RL.txt Eq. (1) for the previous action; par = [T_ref, w1, w2]; e_T is the TRUE error.
reward = -(e_T / par(1))^2 - par(2) * (T_a_prev - T_a_prev2)^2 - par(3) * T_a_prev^2;
isdone = double(abs(e_T) > done_eT);
